simulink model "problem2sml"  (R2023a)
settings: Solver=VariableStepAuto  StartTime=0.0  StopTime=300  RelTol=1e-3
values from neighbouring files (symbols this model uses):
  c1 = 4/(pi*D^2)    (= 0.0127323954474)    [HW1_Group3_2.m]
  c2 = (4*sqrt(p*g))/(Rf*pi*D^2)    [HW1_Group3_2.m]
  c2bar = c2/(2*sqrt(h0))    [HW1_Group3_2.m]
  deltaQ = deltaQ2    (= 1)    [HW1_Group3_2.m]
  h0 = 1    [HW1_Group3_2.m]
  Q0 = sqrt(p*g*h0)/Rf    [HW1_Group3_2.m]
settings Model: Creator=USER  LastModifiedBy=USER

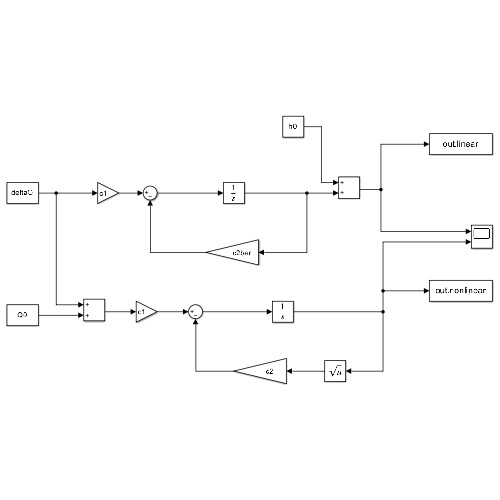
[thumbnail: Simulink's stored preview of the top-level diagram]
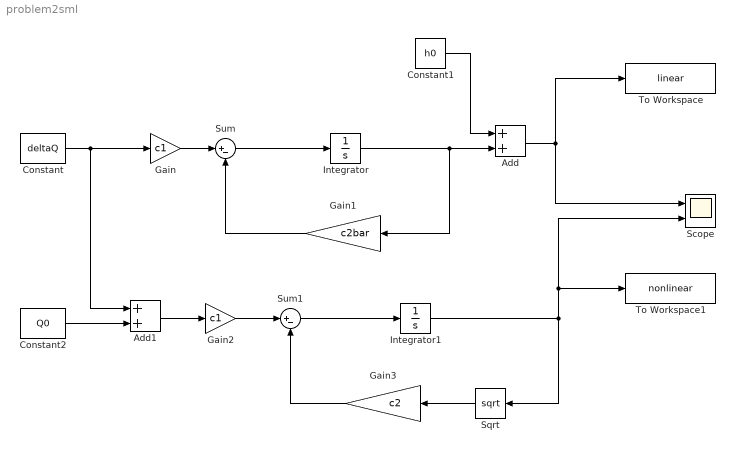
== system problem2sml ==
  Add : Sum
  Add1 : Sum
  Constant : Constant  Value=deltaQ
  Constant1 : Constant  Value=h0
  Constant2 : Constant  Value=Q0
  Gain : Gain  Gain=c1
  Gain1 : Gain  Gain=c2bar
  Gain2 : Gain  Gain=c1
  Gain3 : Gain  Gain=c2
  Integrator : Integrator
  Integrator1 : Integrator  InitialCondition=h0
  Scope : Scope  NumInputPorts=2
  Sqrt : Sqrt
  Sum : Sum  Inputs=|+-
  Sum1 : Sum  Inputs=|+-
  To Workspace : ToWorkspace  VariableName=linear  SaveFormat=Timeseries  SampleTime=-1
  To Workspace1 : ToWorkspace  VariableName=nonlinear  SaveFormat=Timeseries  SampleTime=-1
  wires:
  Constant/1 -> Gain/1, Add1/1
  Gain/1 -> Sum/1
  Sum/1 -> Integrator/1
  Integrator/1 -> Add/2, Gain1/1
  Gain1/1 -> Sum/2
  Constant1/1 -> Add/1
  Add/1 -> To Workspace/1, Scope/1
  Constant2/1 -> Add1/2
  Add1/1 -> Gain2/1
  Gain2/1 -> Sum1/1
  Sum1/1 -> Integrator1/1
  Gain3/1 -> Sum1/2
  Integrator1/1 -> Scope/2, To Workspace1/1, Sqrt/1
  Sqrt/1 -> Gain3/1
